simulink model "modelo1"  (R2016a)
settings: Solver=VariableStepAuto  StartTime=0.0  StopTime=2000  RelTol=1e-3
libraries: simulink x2
settings Model: Creator=Brunno  LastModifiedBy=Brunno

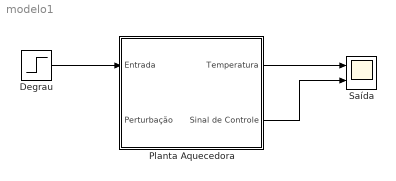
== system modelo1 ==
  Degrau : Step  Time=[1000]  Before=[40]  After=[60]  SampleTime=0
  Planta Aquecedora : Subsystem
  Saída : Scope  NumInputPorts=2
  wires:
  Planta Aquecedora/1(Temperatura) -> Saída/1
  Planta Aquecedora/2(Sinal de Controle) -> Saída/2
  Degrau/1 -> Planta Aquecedora/1(Entrada)

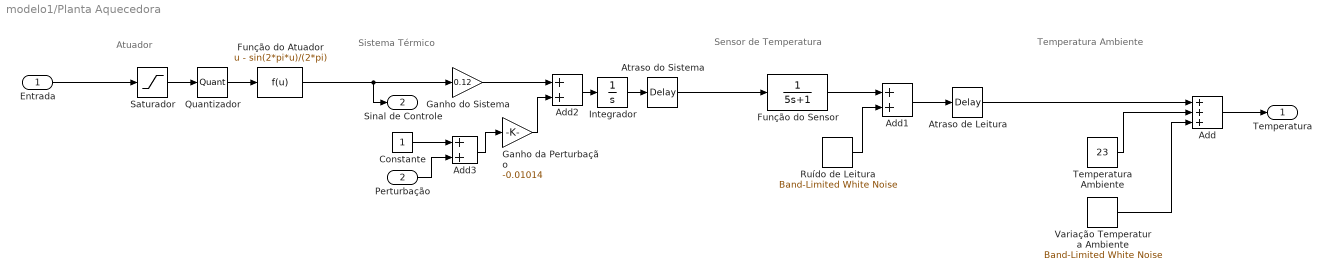
== system modelo1/Planta Aquecedora ==
  note: Temperatura Ambiente
  note: Sistema Térmico
  note: Atuador
  note: Sensor de Temperatura
  Entrada : Inport
  Perturbação : Inport  Port=2
  Add : Sum  Inputs=+++
  Add1 : Sum
  Add2 : Sum
  Add3 : Sum
  Atraso de Leitura : TransportDelay
  Atraso do Sistema : TransportDelay  DelayTime=5
  Constante : Constant
  Função do Atuador : Fcn  Expr=u - sin(2*pi*u)/(2*pi)
  Função do Sensor : TransferFcn  Denominator=[5 1]
  Ganho da Perturbação : Gain  Gain=-0.01014
  Ganho do Sistema : Gain  Gain=0.12
  Integrador : Integrator  LimitOutput=on  UpperSaturationLimit=100 - 23  LowerSaturationLimit=0
  Quantizador : Quantizer  QuantizationInterval=1/255
  Ruído de Leitura : simulink/Sources/Band-Limited White Noise  Cov=[0.05]  Ts=20  seed=[23341]
  Saturador : Saturate  UpperLimit=1  LowerLimit=0
  Temperatura Ambiente : Constant  Value=23
  Variação Temperatura Ambiente : simulink/Sources/Band-Limited White Noise  Cov=[1]  Ts=100  seed=[23341]
  Temperatura : Outport
  Sinal de Controle : Outport  Port=2
  wires:
  Temperatura Ambiente/1 -> Add/2
  Entrada/1 -> Saturador/1
  Integrador/1 -> Atraso do Sistema/1
  Saturador/1 -> Quantizador/1
  Quantizador/1 -> Função do Atuador/1
  Função do Atuador/1 -> Sinal de Controle/1, Ganho do Sistema/1
  Ganho do Sistema/1 -> Add2/1
  Add2/1 -> Integrador/1
  Ganho da Perturbação/1 -> Add2/2
  Variação Temperatura Ambiente/1 -> Add/3
  Atraso do Sistema/1 -> Função do Sensor/1
  Atraso de Leitura/1 -> Add/1
  Add/1 -> Temperatura/1
  Função do Sensor/1 -> Add1/1
  Add1/1 -> Atraso de Leitura/1
  Ruído de Leitura/1 -> Add1/2
  Add3/1 -> Ganho da Perturbação/1
  Constante/1 -> Add3/1
  Perturbação/1 -> Add3/2
